simulink model "ST_ESP_ESM_2017a"  (R2017a)
settings: Solver=ode1  StartTime=0.0  StopTime=SIM_time  FixedStep=stepsize  RelTol=1e-3  EnableMultiTasking=on
undefined symbols (not defined in the file): A, brems_k_max, cw, delta_lr, fah_dkv, fzg_Jz, fzg_l, fzg_lh, fzg_lv, fzg_m, fzg_s, g, h_sp, i_diff, i_getr, i_lenk, init_v0, len_wahl, mue_h, mue_v, omega_max, p_max, rad_r, rho, sin_freq, step_time, sw_ESP
libraries: simulink x2
(part 2 of 2)

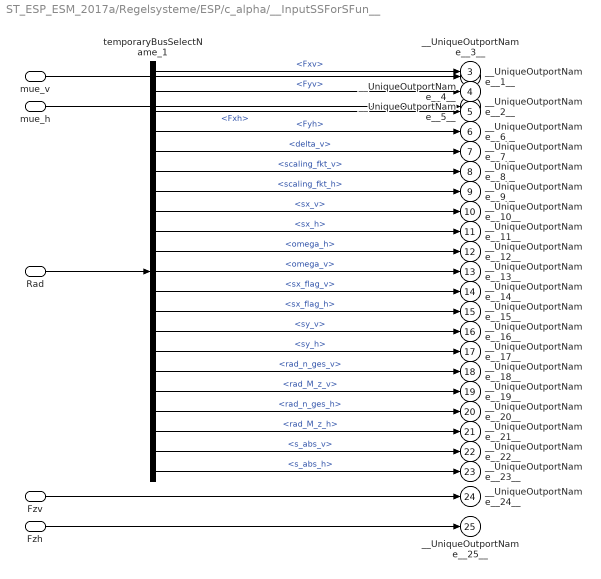
== system ST_ESP_ESM_2017a/Regelsysteme/ESP/c_alpha/__InputSSForSFun__ ==
  mue_v : Inport
  mue_h : Inport  Port=2
  Rad : Inport  Port=3
  Fzv : Inport  Port=4
  Fzh : Inport  Port=5
  temporaryBusSelectName_1 : BusSelector  OutputSignals=Fxv,Fyv,Fxh,Fyh,delta_v,scaling_fkt_v,scaling_fkt_h,sx_v,sx_h,omega_h,omega_v,sx_flag_v,sx_flag_h,sy_v,sy_h,rad_Mz.rad_n_ges_v,rad_Mz.rad_M_z_v,rad_Mz.rad_n_ges_h,rad_Mz.rad_M_z_h,s_abs_v,s_abs_h
  __UniqueOutportName__1__ : Outport
  __UniqueOutportName__2__ : Outport  Port=2
  __UniqueOutportName__3__ : Outport  Port=3
  __UniqueOutportName__4__ : Outport  Port=4
  __UniqueOutportName__5__ : Outport  Port=5
  __UniqueOutportName__6__ : Outport  Port=6
  __UniqueOutportName__7__ : Outport  Port=7
  __UniqueOutportName__8__ : Outport  Port=8
  __UniqueOutportName__9__ : Outport  Port=9
  __UniqueOutportName__10__ : Outport  Port=10
  __UniqueOutportName__11__ : Outport  Port=11
  __UniqueOutportName__12__ : Outport  Port=12
  __UniqueOutportName__13__ : Outport  Port=13
  __UniqueOutportName__14__ : Outport  Port=14
  __UniqueOutportName__15__ : Outport  Port=15
  __UniqueOutportName__16__ : Outport  Port=16
  __UniqueOutportName__17__ : Outport  Port=17
  __UniqueOutportName__18__ : Outport  Port=18
  __UniqueOutportName__19__ : Outport  Port=19
  __UniqueOutportName__20__ : Outport  Port=20
  __UniqueOutportName__21__ : Outport  Port=21
  __UniqueOutportName__22__ : Outport  Port=22
  __UniqueOutportName__23__ : Outport  Port=23
  __UniqueOutportName__24__ : Outport  Port=24
  __UniqueOutportName__25__ : Outport  Port=25
  wires:
  Fzh/1 -> __UniqueOutportName__25__/1
  Fzv/1 -> __UniqueOutportName__24__/1
  temporaryBusSelectName_1/21 -> __UniqueOutportName__23__/1  "<s_abs_h>"
  temporaryBusSelectName_1/20 -> __UniqueOutportName__22__/1  "<s_abs_v>"
  temporaryBusSelectName_1/19 -> __UniqueOutportName__21__/1  "<rad_M_z_h>"
  temporaryBusSelectName_1/18 -> __UniqueOutportName__20__/1  "<rad_n_ges_h>"
  temporaryBusSelectName_1/17 -> __UniqueOutportName__19__/1  "<rad_M_z_v>"
  temporaryBusSelectName_1/16 -> __UniqueOutportName__18__/1  "<rad_n_ges_v>"
  temporaryBusSelectName_1/15 -> __UniqueOutportName__17__/1  "<sy_h>"
  temporaryBusSelectName_1/14 -> __UniqueOutportName__16__/1  "<sy_v>"
  temporaryBusSelectName_1/13 -> __UniqueOutportName__15__/1  "<sx_flag_h>"
  temporaryBusSelectName_1/12 -> __UniqueOutportName__14__/1  "<sx_flag_v>"
  temporaryBusSelectName_1/11 -> __UniqueOutportName__13__/1  "<omega_v>"
  temporaryBusSelectName_1/10 -> __UniqueOutportName__12__/1  "<omega_h>"
  temporaryBusSelectName_1/9 -> __UniqueOutportName__11__/1  "<sx_h>"
  temporaryBusSelectName_1/8 -> __UniqueOutportName__10__/1  "<sx_v>"
  temporaryBusSelectName_1/7 -> __UniqueOutportName__9__/1  "<scaling_fkt_h>"
  temporaryBusSelectName_1/6 -> __UniqueOutportName__8__/1  "<scaling_fkt_v>"
  temporaryBusSelectName_1/5 -> __UniqueOutportName__7__/1  "<delta_v>"
  temporaryBusSelectName_1/4 -> __UniqueOutportName__6__/1  "<Fyh>"
  temporaryBusSelectName_1/3 -> __UniqueOutportName__5__/1  "<Fxh>"
  temporaryBusSelectName_1/2 -> __UniqueOutportName__4__/1  "<Fyv>"
  temporaryBusSelectName_1/1 -> __UniqueOutportName__3__/1  "<Fxv>"
  mue_h/1 -> __UniqueOutportName__2__/1
  mue_v/1 -> __UniqueOutportName__1__/1
  Rad/1 -> temporaryBusSelectName_1/1

== system ST_ESP_ESM_2017a/Regelsysteme/ESP/c_alpha/__OutputSSForSFun__ ==
  __UniqueInportName__1__ : Inport
  __UniqueInportName__2__ : Inport  Port=2
  c_alpha_v : Outport
  c_alpha_h : Outport  Port=2
  wires:
  __UniqueInportName__2__/1 -> c_alpha_h/1
  __UniqueInportName__1__/1 -> c_alpha_v/1

== matlab function ST_ESP_ESM_2017a/Regelsysteme/ESP/Implementierung PID-Regler/D-Anteil ==
  data: y output; delta_psi_p input; v input
function y = fcn(delta_psi_p, v)
if v<=70
    Faktor=-1/70.*v+1;
else
    Faktor=0;
end   
gain=1;
y = gain*Faktor*delta_psi_p;

== matlab function ST_ESP_ESM_2017a/Regelsysteme/ESP/Implementierung PID-Regler/P-Anteil ==
  data: beta input; delta_psi_p input; y output; v input
function y = fcn(beta,delta_psi_p, v)
if v<=70
    Faktor=-1/70.*v+1;
else
    Faktor=0;
end    
gain=2500;
y = gain*(Faktor*sign(beta)*sqrt(abs(beta))+Faktor*delta_psi_p);

== matlab function ST_ESP_ESM_2017a/Regelsysteme/ESP/Implementierung PID-Regler/I-Anteil ==
  data: delta_psi_p input; y output; v input
function y = fcn(delta_psi_p, v)
if v<=70
    Faktor=-1/70.*v+1;
else
    Faktor=0;
end 
gain=250;
y = gain*Faktor*delta_psi_p;

== matlab function ST_ESP_ESM_2017a/Regelsysteme/ESP/Implementierung PID-Regler/Dead Zone ==
  data: u input; y output
function y = fcn(u)
deadpoint=100;
if u>deadpoint||u<-deadpoint
    y=u;
else
    y=0;
end
